simulink model "HybridControllerD3D3_nAct"  (Simulink 7.5)
settings: Solver=FixedStepDiscrete  StartTime=0.0  StopTime=inf  RelTol=1e-3
PreLoadFcn:
  | initializeSimulation
values from neighbouring files (symbols this model uses):
  nAct = 8    [initializeSimulation.m]
  nDout = 4    [initializeSimulation.m]
  node = completenodestruct(node)    [initializeSimulation.m]
undefined symbols (not defined in the file or in its folder): HybridCtrlParameters
libraries: xpclib x14, xpcsystranlib x8, simulink x4
CloseFcn:
  | rtwprivate ssgencode ModelCloseRequest scrnet_receiver
settings Model: Creator=mvetsch  LastModifiedBy=Andreas  ExtModeArmWhenConnect=off  BufferReuse=off
settings DataIOCC: LimitDataPoints=off  SaveOutput=off  SignalLogging=off  SaveTime=off  SignalLoggingName=sigsOut
settings OptimizationCC: BlockReduction=off  OptimizeBlockIOStorage=off  BufferReuse=off  EnforceIntegerDowncast=off  ExpressionFolding=off  FoldNonRolledExpr=off  LocalBlockOutputs=off  StateBitsets=on  DataBitsets=on  UseTempVars=on  InitFltsAndDblsToZero=on  EfficientFloat2IntCast=on  SimCompilerOptimization=On
settings DebuggingCC: SaveWithParameterizedLinksMsg=none  CheckSSInitialOutputMsg=off  SolverPrmCheckMsg=none  StrictBusMsg=None
settings HardwareCC: ProdIntDivRoundTo=Zero  ProdEndianess=LittleEndian  ProdHWDeviceType=Generic->32-bit x86 compatible  TargetHWDeviceType=32-bit Generic
settings SFSimCC: SimCustomHeaderCode="#include \"PredictorCorrector.h\""  SimUserSources=PredictorCorrector.c  SimUserIncludeDirs=D:\PredictorCorrector\HybridSimToolbox
settings RTWCC: SystemTargetFile=xpctarget.tlc  TemplateMakefile=xpc_default_tmf  Description=xPC Target  ProcessScript=xpctarget_make_rtw_hook  CustomHeaderCode="#include \"PredictorCorrector.h\""  CustomInclude=D:\PredictorCorrector\HybridSimToolbox  CustomSource=PredictorCorrector.c  IncludeERTFirstTime=on  RTWCompilerOptimization=On
settings xpcTargetCC: TargetFcnLib=ansi_tfl_tmw.mat  TargetFunctionLibrary=ANSI_C  ERTCodeCoverageTool=None  ParMdlRefBuildCompliant=off  PortableWordSizes=off  RL32IRQSourceModifier=11  xPCIRQSourceBoard=Scramnet_SC150+  xPCLoadParamSetFile=off

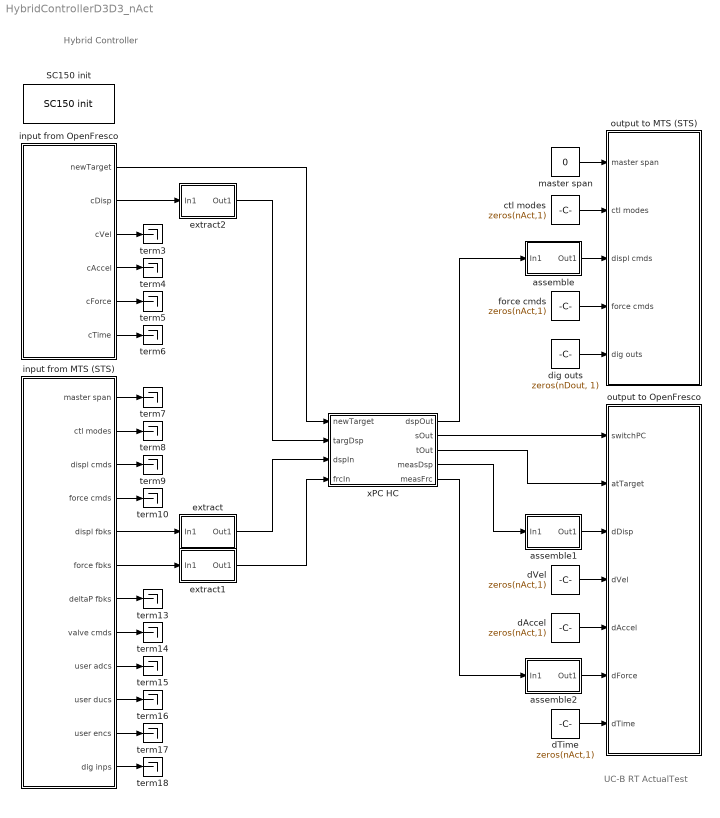
== system HybridControllerD3D3_nAct ==
  note: Hybrid Controller
  note: UC-B RT ActualTest
  SC150 init : xpcsystranlib/Shared Memory/SC150 init   node=node  pci=-1
  assemble : Subsystem  mask(to Actuators){id=[2 3 4 1 5 6], size=nAct}
      mask prompts: id "Index Vector: id"; size "Vector Size: size"
      mask help: To select to which actuator(s) the signals are going to
      mask Display: disp('Assemble')
  assemble1 : Subsystem  mask(to Actuators){id=[2 3 4 1 5 6], size=nAct}
      mask prompts: id "Index Vector: id"; size "Vector Size: size"
      mask help: To select to which actuator(s) the signals are going to
      mask Display: disp('Assemble')
  assemble2 : Subsystem  mask(to Actuators){id=[2 3 4 1 5 6], size=nAct}
      mask prompts: id "Index Vector: id"; size "Vector Size: size"
      mask help: To select to which actuator(s) the signals are going to
      mask Display: disp('Assemble')
  ctl modes : Constant  Value=zeros(nAct,1)  OutDataType=sfix(16)  OutScaling=2^0
  dAccel : Constant  Value=zeros(nAct,1)  OutDataType=sfix(16)  OutScaling=2^0
  dTime : Constant  Value=zeros(nAct,1)  OutDataType=sfix(16)  OutScaling=2^0
  dVel : Constant  Value=zeros(nAct,1)  OutDataType=sfix(16)  OutScaling=2^0
  dig outs : Constant  Value=zeros(nDout, 1)  OutDataTypeMode=uint32  OutDataType=sfix(16)  OutScaling=2^0  OutDataTypeStr=uint32
  extract : Subsystem  mask(from Actuators){id=[2 3 4 1 5 6], size=nAct}
      mask prompts: id "Index Vector: id"; size "Vector Size: size"
      mask help: To select from which actuator(s) the signals are coming from
      mask Display: disp('Extract')
  extract1 : Subsystem  mask(from Actuators){id=[2 3 4 1 5 6], size=nAct}
      mask prompts: id "Index Vector: id"; size "Vector Size: size"
      mask help: To select from which actuator(s) the signals are coming from
      mask Display: disp('Extract')
  extract2 : Subsystem  mask(from Actuators){id=[2 3 4 1 5 6], size=nAct}
      mask prompts: id "Index Vector: id"; size "Vector Size: size"
      mask help: To select from which actuator(s) the signals are coming from
      mask Display: disp('Extract')
  force cmds : Constant  Value=zeros(nAct,1)  OutDataType=sfix(16)  OutScaling=2^0
  input from MTS (STS) : Subsystem
  input from OpenFresco : Subsystem
  master span : Constant  Value=0  OutDataType=sfix(16)  OutScaling=2^0
  output to MTS (STS) : Subsystem
  output to OpenFresco : Subsystem
  term{3..10,13..18} (14 alike) : Terminator
  xPC HC : Subsystem  mask(Hybrid Controller: D3/D3){nAct=6, dtInt=HybridCtrlParameters.dtInt, dtSim=HybridCtrlParameters.dtSim, dtCon=HybridCtrlParameters.dtCon, N=HybridCtrlParameters.N, iDelay=HybridCtrlParameters.iDelay}
      mask prompts: nAct "Number of Actuators: nAct"; dtInt "Integration time step: dtInt"; dtSim "Simulation time step: dtSim"; dtCon "Controller time step: dtCon"; N "Maximum number of substeps: N"; iDelay "Number of delay steps: iDelay"
      mask help: Hybrid Controller using C0-continuous cubic Lagrange interpolation for prediction and correction
      mask Display: disp('xPC Target\nHybrid Controller\n(D3/D3)')
  wires:
  input from MTS (STS)/10(user ducs) -> term16/1
  input from MTS (STS)/12(dig inps) -> term18/1
  input from MTS (STS)/2(ctl modes) -> term8/1
  input from MTS (STS)/4(force cmds) -> term10/1
  input from MTS (STS)/8(valve cmds) -> term14/1
  input from MTS (STS)/1(master span) -> term7/1
  input from MTS (STS)/7(deltaP fbks) -> term13/1
  input from MTS (STS)/9(user adcs) -> term15/1
  input from MTS (STS)/11(user encs) -> term17/1
  master span/1 -> output to MTS (STS)/1(master span)
  force cmds/1 -> output to MTS (STS)/4(force cmds)
  ctl modes/1 -> output to MTS (STS)/2(ctl modes)
  input from MTS (STS)/3(displ cmds) -> term9/1
  input from MTS (STS)/5(displ fbks) -> extract/1(In1)
  dig outs/1 -> output to MTS (STS)/5(dig outs)
  input from MTS (STS)/6(force fbks) -> extract1/1(In1)
  dVel/1 -> output to OpenFresco/4(dVel)
  dAccel/1 -> output to OpenFresco/5(dAccel)
  dTime/1 -> output to OpenFresco/7(dTime)
  input from OpenFresco/3(cVel) -> term3/1
  input from OpenFresco/4(cAccel) -> term4/1
  input from OpenFresco/5(cForce) -> term5/1
  input from OpenFresco/6(cTime) -> term6/1
  assemble/1(Out1) -> output to MTS (STS)/3(displ cmds)
  input from OpenFresco/2(cDisp) -> extract2/1(In1)
  input from OpenFresco/1(newTarget) -> xPC HC/1(newTarget)
  extract2/1(Out1) -> xPC HC/2(targDsp)
  extract/1(Out1) -> xPC HC/3(dspIn)
  extract1/1(Out1) -> xPC HC/4(frcIn)
  xPC HC/1(dspOut) -> assemble/1(In1)
  xPC HC/5(measFrc) -> assemble2/1(In1)
  xPC HC/4(measDsp) -> assemble1/1(In1)
  xPC HC/3(tOut) -> output to OpenFresco/2(atTarget)
  xPC HC/2(sOut) -> output to OpenFresco/1(switchPC)
  assemble1/1(Out1) -> output to OpenFresco/3(dDisp)
  assemble2/1(Out1) -> output to OpenFresco/6(dForce)

== system HybridControllerD3D3_nAct/assemble ==
  In1 : Inport  OutDataType=sfix(16)  OutScaling=2^0
  Assignment : Assignment  OutputInitialize=Specify size for each dimension in table  IndexOptions=Index vector (port)  Indices=1  OutputSizes=nAct
  Constant : Constant  Value=id  OutDataType=sfix(16)  OutScaling=2^0
  Out1 : Outport  OutDataType=sfix(16)  OutScaling=2^0
  wires:
  Constant/1 -> Assignment/2
  Assignment/1 -> Out1/1
  In1/1 -> Assignment/1

== system HybridControllerD3D3_nAct/assemble1 ==
  In1 : Inport  OutDataType=sfix(16)  OutScaling=2^0
  Assignment : Assignment  OutputInitialize=Specify size for each dimension in table  IndexOptions=Index vector (port)  Indices=1  OutputSizes=nAct
  Constant : Constant  Value=id  OutDataType=sfix(16)  OutScaling=2^0
  Out1 : Outport  OutDataType=sfix(16)  OutScaling=2^0
  wires:
  Constant/1 -> Assignment/2
  Assignment/1 -> Out1/1
  In1/1 -> Assignment/1

== system HybridControllerD3D3_nAct/assemble2 ==
  In1 : Inport  OutDataType=sfix(16)  OutScaling=2^0
  Assignment : Assignment  OutputInitialize=Specify size for each dimension in table  IndexOptions=Index vector (port)  Indices=1  OutputSizes=nAct
  Constant : Constant  Value=id  OutDataType=sfix(16)  OutScaling=2^0
  Out1 : Outport  OutDataType=sfix(16)  OutScaling=2^0
  wires:
  Constant/1 -> Assignment/2
  Assignment/1 -> Out1/1
  In1/1 -> Assignment/1

== system HybridControllerD3D3_nAct/extract ==
  In1 : Inport  OutDataType=sfix(16)  OutScaling=2^0
  Selector : Selector  InputPortWidth=size  IndexOptions=Index vector (dialog)  Indices=id  OutputSizes=1
  Out1 : Outport  OutDataType=sfix(16)  OutScaling=2^0
  wires:
  Selector/1 -> Out1/1
  In1/1 -> Selector/1

== system HybridControllerD3D3_nAct/extract1 ==
  In1 : Inport  OutDataType=sfix(16)  OutScaling=2^0
  Selector : Selector  InputPortWidth=size  IndexOptions=Index vector (dialog)  Indices=id  OutputSizes=1
  Out1 : Outport  OutDataType=sfix(16)  OutScaling=2^0
  wires:
  Selector/1 -> Out1/1
  In1/1 -> Selector/1

== system HybridControllerD3D3_nAct/extract2 ==
  In1 : Inport  OutDataType=sfix(16)  OutScaling=2^0
  Selector : Selector  InputPortWidth=size  IndexOptions=Index vector (dialog)  Indices=id  OutputSizes=1
  Out1 : Outport  OutDataType=sfix(16)  OutScaling=2^0
  wires:
  Selector/1 -> Out1/1
  In1/1 -> Selector/1

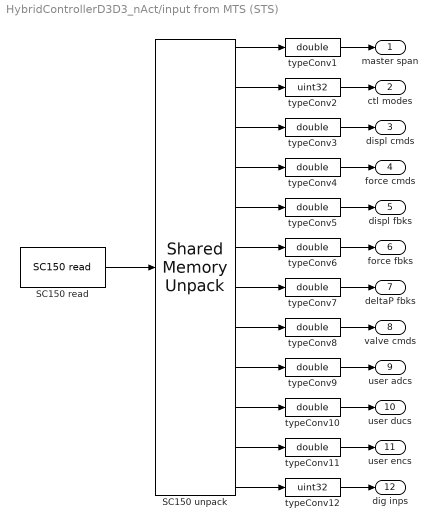
== system HybridControllerD3D3_nAct/input from MTS (STS) ==
  SC150 read : xpcsystranlib/Shared Memory/SC150 read   partition=node.Partitions(12:23)  errorport=off  ts=samplePeriod  pci=-1
  SC150 unpack : xpclib/Shared Memory/Shared Memory Unpack   partition=node.Partitions(12:23)
  typeConv{1,3..11} (10 alike) : DataTypeConversion  OutDataTypeMode=double  OutDataType=sfix(16)  OutScaling=2^0  OutDataTypeStr=double  SaturateOnIntegerOverflow=on  RndMeth=Zero
  typeConv12 : DataTypeConversion  OutDataTypeMode=uint32  OutDataType=sfix(16)  OutScaling=2^0  OutDataTypeStr=uint32  SaturateOnIntegerOverflow=on  RndMeth=Zero
  typeConv2 : DataTypeConversion  OutDataTypeMode=uint32  OutDataType=sfix(16)  OutScaling=2^0  OutDataTypeStr=uint32  SaturateOnIntegerOverflow=on  RndMeth=Zero
  master span : Outport  OutDataType=sfix(16)  OutScaling=2^0
  ctl modes : Outport  Port=2  OutDataType=sfix(16)  OutScaling=2^0
  displ cmds : Outport  Port=3  OutDataType=sfix(16)  OutScaling=2^0
  force cmds : Outport  Port=4  OutDataType=sfix(16)  OutScaling=2^0
  displ fbks : Outport  Port=5  OutDataType=sfix(16)  OutScaling=2^0
  force fbks : Outport  Port=6  OutDataType=sfix(16)  OutScaling=2^0
  deltaP fbks : Outport  Port=7  OutDataType=sfix(16)  OutScaling=2^0
  valve cmds : Outport  Port=8  OutDataType=sfix(16)  OutScaling=2^0
  user adcs : Outport  Port=9  OutDataType=sfix(16)  OutScaling=2^0
  user ducs : Outport  Port=10  OutDataType=sfix(16)  OutScaling=2^0
  user encs : Outport  Port=11  OutDataType=sfix(16)  OutScaling=2^0
  dig inps : Outport  Port=12  OutDataType=sfix(16)  OutScaling=2^0
  wires:
  typeConv11/1 -> user encs/1
  typeConv10/1 -> user ducs/1
  typeConv12/1 -> dig inps/1
  typeConv9/1 -> user adcs/1
  typeConv8/1 -> valve cmds/1
  typeConv7/1 -> deltaP fbks/1
  typeConv6/1 -> force fbks/1
  typeConv5/1 -> displ fbks/1
  typeConv4/1 -> force cmds/1
  typeConv3/1 -> displ cmds/1
  typeConv1/1 -> master span/1
  SC150 read/1 -> SC150 unpack/1
  typeConv2/1 -> ctl modes/1
  SC150 unpack/1 -> typeConv1/1
  SC150 unpack/2 -> typeConv2/1
  SC150 unpack/3 -> typeConv3/1
  SC150 unpack/4 -> typeConv4/1
  SC150 unpack/5 -> typeConv5/1
  SC150 unpack/6 -> typeConv6/1
  SC150 unpack/7 -> typeConv7/1
  SC150 unpack/8 -> typeConv8/1
  SC150 unpack/9 -> typeConv9/1
  SC150 unpack/10 -> typeConv10/1
  SC150 unpack/11 -> typeConv11/1
  SC150 unpack/12 -> typeConv12/1

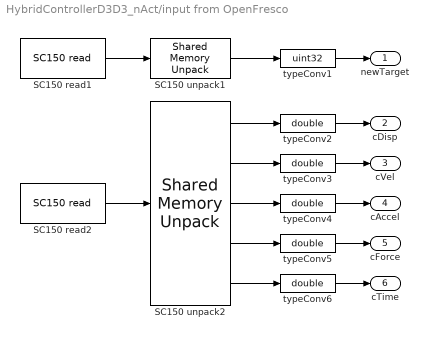
== system HybridControllerD3D3_nAct/input from OpenFresco ==
  SC150 read1 : xpcsystranlib/Shared Memory/SC150 read   partition=node.Partitions(26)  errorport=off  ts=samplePeriod  pci=-1
  SC150 read2 : xpcsystranlib/Shared Memory/SC150 read   partition=node.Partitions(29:33)  errorport=off  ts=samplePeriod  pci=-1
  SC150 unpack1 : xpclib/Shared Memory/Shared Memory Unpack   partition=node.Partitions(26)
  SC150 unpack2 : xpclib/Shared Memory/Shared Memory Unpack   partition=node.Partitions(29:33)
  typeConv1 : DataTypeConversion  OutDataTypeMode=uint32  OutDataType=sfix(16)  OutScaling=2^0  OutDataTypeStr=uint32  SaturateOnIntegerOverflow=on  RndMeth=Zero
  typeConv{2..6} (5 alike) : DataTypeConversion  OutDataTypeMode=double  OutDataType=sfix(16)  OutScaling=2^0  OutDataTypeStr=double  SaturateOnIntegerOverflow=on  RndMeth=Zero
  newTarget : Outport  OutDataType=sfix(16)  OutScaling=2^0
  cDisp : Outport  Port=2  OutDataType=sfix(16)  OutScaling=2^0
  cVel : Outport  Port=3  OutDataType=sfix(16)  OutScaling=2^0
  cAccel : Outport  Port=4  OutDataType=sfix(16)  OutScaling=2^0
  cForce : Outport  Port=5  OutDataType=sfix(16)  OutScaling=2^0
  cTime : Outport  Port=6  OutDataType=sfix(16)  OutScaling=2^0
  wires:
  typeConv1/1 -> newTarget/1
  SC150 read1/1 -> SC150 unpack1/1
  SC150 unpack1/1 -> typeConv1/1
  typeConv2/1 -> cDisp/1
  SC150 unpack2/1 -> typeConv2/1
  typeConv3/1 -> cVel/1
  SC150 unpack2/2 -> typeConv3/1
  typeConv4/1 -> cAccel/1
  SC150 unpack2/3 -> typeConv4/1
  typeConv5/1 -> cForce/1
  typeConv6/1 -> cTime/1
  SC150 unpack2/5 -> typeConv6/1
  SC150 read2/1 -> SC150 unpack2/1
  SC150 unpack2/4 -> typeConv5/1

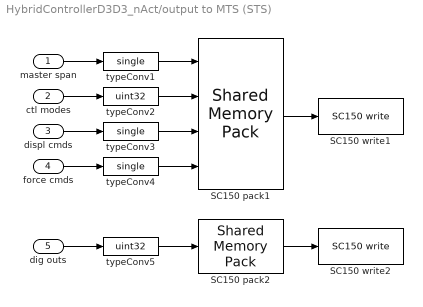
== system HybridControllerD3D3_nAct/output to MTS (STS) ==
  master span : Inport  OutDataType=sfix(16)  OutScaling=2^0
  ctl modes : Inport  Port=2  OutDataType=sfix(16)  OutScaling=2^0
  displ cmds : Inport  Port=3  OutDataType=sfix(16)  OutScaling=2^0
  force cmds : Inport  Port=4  OutDataType=sfix(16)  OutScaling=2^0
  dig outs : Inport  Port=5  OutDataType=sfix(16)  OutScaling=2^0
  SC150 pack1 : xpclib/Shared Memory/Shared Memory Pack   partition=node.Partitions(1:4)
  SC150 pack2 : xpclib/Shared Memory/Shared Memory Pack   partition=node.Partitions(11)
  SC150 write1 : xpcsystranlib/Shared Memory/SC150 write   partition=node.Partitions(1:4)  errorport=off  ts=samplePeriod  pci=-1
  SC150 write2 : xpcsystranlib/Shared Memory/SC150 write   partition=node.Partitions(11)  errorport=off  ts=samplePeriod  pci=-1
  typeConv1 : DataTypeConversion  OutDataTypeMode=single  OutDataType=sfix(16)  OutScaling=2^0  OutDataTypeStr=single  SaturateOnIntegerOverflow=on  RndMeth=Zero
  typeConv2 : DataTypeConversion  OutDataTypeMode=uint32  OutDataType=sfix(16)  OutScaling=2^0  OutDataTypeStr=uint32  SaturateOnIntegerOverflow=on  RndMeth=Zero
  typeConv3 : DataTypeConversion  OutDataTypeMode=single  OutDataType=sfix(16)  OutScaling=2^0  OutDataTypeStr=single  SaturateOnIntegerOverflow=on  RndMeth=Zero
  typeConv4 : DataTypeConversion  OutDataTypeMode=single  OutDataType=sfix(16)  OutScaling=2^0  OutDataTypeStr=single  SaturateOnIntegerOverflow=on  RndMeth=Zero
  typeConv5 : DataTypeConversion  OutDataTypeMode=uint32  OutDataType=sfix(16)  OutScaling=2^0  OutDataTypeStr=uint32  SaturateOnIntegerOverflow=on  RndMeth=Zero
  wires:
  dig outs/1 -> typeConv5/1
  force cmds/1 -> typeConv4/1
  master span/1 -> typeConv1/1
  SC150 pack1/1 -> SC150 write1/1
  displ cmds/1 -> typeConv3/1
  ctl modes/1 -> typeConv2/1
  typeConv1/1 -> SC150 pack1/1
  typeConv2/1 -> SC150 pack1/2
  typeConv3/1 -> SC150 pack1/3
  typeConv4/1 -> SC150 pack1/4
  SC150 pack2/1 -> SC150 write2/1
  typeConv5/1 -> SC150 pack2/1

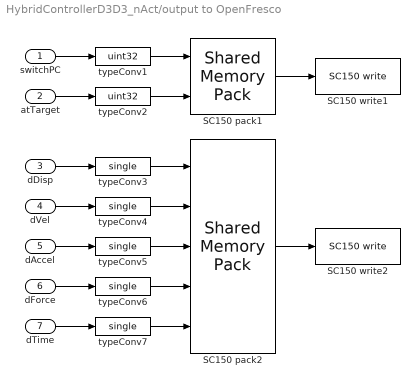
== system HybridControllerD3D3_nAct/output to OpenFresco ==
  switchPC : Inport  OutDataType=sfix(16)  OutScaling=2^0
  atTarget : Inport  Port=2  OutDataType=sfix(16)  OutScaling=2^0
  dDisp : Inport  Port=3  OutDataType=sfix(16)  OutScaling=2^0
  dVel : Inport  Port=4  OutDataType=sfix(16)  OutScaling=2^0
  dAccel : Inport  Port=5  OutDataType=sfix(16)  OutScaling=2^0
  dForce : Inport  Port=6  OutDataType=sfix(16)  OutScaling=2^0
  dTime : Inport  Port=7  OutDataType=sfix(16)  OutScaling=2^0
  SC150 pack1 : xpclib/Shared Memory/Shared Memory Pack   partition=node.Partitions(27:28)
  SC150 pack2 : xpclib/Shared Memory/Shared Memory Pack   partition=node.Partitions(34:38)
  SC150 write1 : xpcsystranlib/Shared Memory/SC150 write   partition=node.Partitions(27:28)  errorport=off  ts=samplePeriod  pci=-1
  SC150 write2 : xpcsystranlib/Shared Memory/SC150 write   partition=node.Partitions(34:38)  errorport=off  ts=samplePeriod  pci=-1
  typeConv1 : DataTypeConversion  OutDataTypeMode=uint32  OutDataType=sfix(16)  OutScaling=2^0  OutDataTypeStr=uint32  SaturateOnIntegerOverflow=on  RndMeth=Zero
  typeConv2 : DataTypeConversion  OutDataTypeMode=uint32  OutDataType=sfix(16)  OutScaling=2^0  OutDataTypeStr=uint32  SaturateOnIntegerOverflow=on  RndMeth=Zero
  typeConv{3..7} (5 alike) : DataTypeConversion  OutDataTypeMode=single  OutDataType=sfix(16)  OutScaling=2^0  OutDataTypeStr=single  SaturateOnIntegerOverflow=on  RndMeth=Zero
  wires:
  dAccel/1 -> typeConv5/1
  switchPC/1 -> typeConv1/1
  SC150 pack1/1 -> SC150 write1/1
  dVel/1 -> typeConv4/1
  dDisp/1 -> typeConv3/1
  typeConv3/1 -> SC150 pack2/1
  typeConv4/1 -> SC150 pack2/2
  typeConv5/1 -> SC150 pack2/3
  dForce/1 -> typeConv6/1
  typeConv6/1 -> SC150 pack2/4
  dTime/1 -> typeConv7/1
  typeConv7/1 -> SC150 pack2/5
  atTarget/1 -> typeConv2/1
  typeConv2/1 -> SC150 pack1/2
  typeConv1/1 -> SC150 pack1/1
  SC150 pack2/1 -> SC150 write2/1

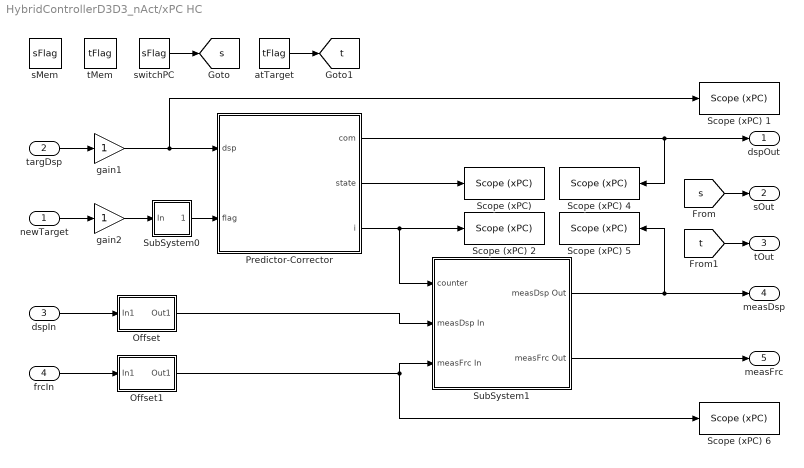
== system HybridControllerD3D3_nAct/xPC HC ==
  newTarget : Inport  OutDataType=sfix(16)  OutScaling=2^0
  targDsp : Inport  Port=2  OutDataType=sfix(16)  OutScaling=2^0
  dspIn : Inport  Port=3  OutDataType=sfix(16)  OutScaling=2^0
  frcIn : Inport  Port=4  OutDataType=sfix(16)  OutScaling=2^0
  Offset : Subsystem  mask(Signal Offset){nS=nAct, nOffset=1024, dt=dtCon}
      mask prompts: nS "Number of Signals: nS"; nOffset "Number of samples to initialize offset: nOffset"; dt "Sample time: dt"
      mask help: Offset signal by average of signal over initial number of samples
      mask Display: fprintf('Signal\nOffset')
  Offset1 : Subsystem  mask(Signal Offset){nS=nAct, nOffset=1024, dt=dtCon}
      mask prompts: nS "Number of Signals: nS"; nOffset "Number of samples to initialize offset: nOffset"; dt "Sample time: dt"
      mask help: Offset signal by average of signal over initial number of samples
      mask Display: fprintf('Signal\nOffset')
  Predictor-Corrector : Stateflow chart  TreatAsAtomicUnit=on
  "Scope (xPC) " : xpclib/Misc./Scope (xPC)   SystemSampleTime=-1  scopeno=4  scopetype=File  autostart=on  viewmode=Graphical redraw  formatstr='%15.6f'  grid=on  ylimits=[0,3]  nosamples=4096  noprepostsamples=0  interleave=1  triggermode=FreeRun  triggersignal=1  triggerlevel=0.0  triggerslope=Either  triggerscope=1  triggersample=0  filename=state.dat  mode=Lazy  writesize=512  autorestart=on  dynamicfilemode=off  maxwritefilesize=512*1024^2
  Scope (xPC) 1 : xpclib/Misc./Scope (xPC)   SystemSampleTime=-1  scopeno=1  scopetype=File  autostart=on  viewmode=Numerical  formatstr='%15.6f'  grid=on  ylimits=[-4,4]  nosamples=4096  noprepostsamples=0  interleave=1  triggermode=FreeRun  triggersignal=1  triggerlevel=0.0  triggerslope=Either  triggerscope=1  triggersample=0  filename=targDsp.dat  mode=Lazy  writesize=512  autorestart=on  dynamicfilemode=off  maxwritefilesize=512*1024^2
  Scope (xPC) 2 : xpclib/Misc./Scope (xPC)   SystemSampleTime=-1  scopeno=5  scopetype=File  autostart=on  viewmode=Numerical  formatstr='%15.6f'  grid=on  ylimits=[0,3]  nosamples=4096  noprepostsamples=0  interleave=1  triggermode=FreeRun  triggersignal=1  triggerlevel=0.0  triggerslope=Either  triggerscope=1  triggersample=0  filename=count.dat  mode=Lazy  writesize=512  autorestart=on  dynamicfilemode=off  maxwritefilesize=512*1024^2
  Scope (xPC) 4 : xpclib/Misc./Scope (xPC)   SystemSampleTime=-1  scopeno=2  scopetype=File  autostart=on  viewmode=Numerical  formatstr='%15.6f'  grid=on  ylimits=[-4,4]  nosamples=4096  noprepostsamples=0  interleave=1  triggermode=FreeRun  triggersignal=1  triggerlevel=0.0  triggerslope=Either  triggerscope=1  triggersample=0  filename=commDsp.dat  mode=Lazy  writesize=512  autorestart=on  dynamicfilemode=off  maxwritefilesize=512*1024^2
  Scope (xPC) 5 : xpclib/Misc./Scope (xPC)   SystemSampleTime=-1  scopeno=3  scopetype=File  autostart=on  viewmode=Numerical  formatstr='%15.6f'  grid=on  ylimits=[-4,4]  nosamples=4096  noprepostsamples=0  interleave=1  triggermode=FreeRun  triggersignal=1  triggerlevel=0.0  triggerslope=Either  triggerscope=1  triggersample=0  filename=measDsp.dat  mode=Lazy  writesize=512  autorestart=on  dynamicfilemode=off  maxwritefilesize=512*1024^2
  Scope (xPC) 6 : xpclib/Misc./Scope (xPC)   SystemSampleTime=-1  scopeno=6  scopetype=File  autostart=on  viewmode=Numerical  formatstr='%15.6f'  grid=on  ylimits=[0,3]  nosamples=4096  noprepostsamples=0  interleave=1  triggermode=FreeRun  triggersignal=1  triggerlevel=0.0  triggerslope=Either  triggerscope=1  triggersample=0  filename=measFrc.dat  mode=Lazy  writesize=512  autorestart=on  dynamicfilemode=off  maxwritefilesize=512*1024^2
  SubSystem0 : Subsystem
  SubSystem1 : Subsystem
  atTarget : DataStoreRead  DataStoreName=tFlag  SampleTime=dtCon
  gain1 : Gain  ParameterDataType=sfix(16)  ParameterScaling=2^0  OutDataType=sfix(16)  OutScaling=2^0
  gain2 : Gain  ParameterDataType=sfix(16)  ParameterScaling=2^0  OutDataType=sfix(16)  OutScaling=2^0  OutDataTypeStr=Inherit: Same as input  ParamDataTypeStr=Inherit: Same as input
  sMem : DataStoreMemory  DataStoreName=sFlag  DataType=uint32  OutDataType=sfix(16)  OutScaling=2^0  OutDataTypeStr=uint32
  switchPC : DataStoreRead  DataStoreName=sFlag  SampleTime=dtCon
  tMem : DataStoreMemory  DataStoreName=tFlag  DataType=uint32  OutDataType=sfix(16)  OutScaling=2^0  OutDataTypeStr=uint32
  dspOut : Outport  OutDataType=sfix(16)  OutScaling=2^0
  sOut : Outport  Port=2  OutDataType=sfix(16)  OutScaling=2^0
  tOut : Outport  Port=3  OutDataType=sfix(16)  OutScaling=2^0
  measDsp : Outport  Port=4  OutDataType=sfix(16)  OutScaling=2^0
  measFrc : Outport  Port=5  OutDataType=sfix(16)  OutScaling=2^0
  tag scope: s=global, t=global
  wires:
  frcIn/1 -> Offset1/1(In1)
  dspIn/1 -> Offset/1(In1)
  SubSystem1/2(measFrc Out) -> measFrc/1
  SubSystem1/1(measDsp Out) -> Scope (xPC) 5/1, measDsp/1
  Predictor-Corrector/3(i) -> SubSystem1/1(counter), Scope (xPC) 2/1
  Predictor-Corrector/2(state) -> "Scope (xPC) "/1
  Predictor-Corrector/1(com) -> dspOut/1, Scope (xPC) 4/1
  Offset/1(Out1) -> SubSystem1/2(measDsp In)
  SubSystem0/1(Out) -> Predictor-Corrector/2(flag)
  newTarget/1 -> gain2/1
  switchPC/1 -> [s]
  atTarget/1 -> [t]
  targDsp/1 -> gain1/1
  Offset1/1(Out1) -> Scope (xPC) 6/1, SubSystem1/3(measFrc In)
  [s] -> sOut/1
  [t] -> tOut/1
  gain1/1 -> Predictor-Corrector/1(dsp), Scope (xPC) 1/1
  gain2/1 -> SubSystem0/1(In)

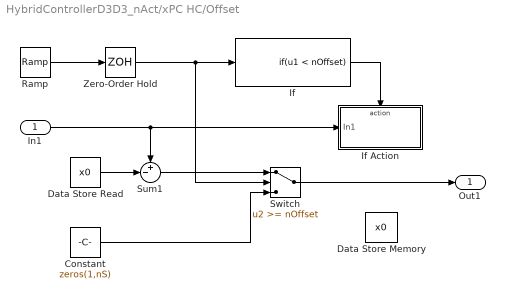
== system HybridControllerD3D3_nAct/xPC HC/Offset ==
  In1 : Inport  OutDataType=sfix(16)  OutScaling=2^0
  Constant : Constant  Value=zeros(1,nS)  OutDataType=sfix(16)  OutScaling=2^0
  Data Store Memory : DataStoreMemory  DataStoreName=x0  InitialValue=zeros(1,nS)  DataType=double  OutDataType=sfix(16)  OutScaling=2^0  OutDataTypeStr=double
  Data Store Read : DataStoreRead  DataStoreName=x0  SampleTime=dt
  If : If  IfExpression=u1 < nOffset  ShowElse=off
  If Action : Subsystem  TreatAsAtomicUnit=on
  Ramp : simulink/Sources/Ramp  SystemSampleTime=-1  slope=1/dt  start=0  X0=0
  Sum1 : Sum  Inputs=+-|  OutDataType=sfix(16)  OutScaling=2^0  SaturateOnIntegerOverflow=on  InputSameDT=on  OutDataTypeStr=Inherit: Same as first input
  Switch : Switch  Threshold=nOffset  SaturateOnIntegerOverflow=on  InputSameDT=on
  Zero-Order Hold : ZeroOrderHold  SampleTime=dt
  Out1 : Outport  OutDataType=sfix(16)  OutScaling=2^0
  wires:
  Switch/1 -> Out1/1
  Sum1/1 -> Switch/1
  Data Store Read/1 -> Sum1/2
  In1/1 -> If Action/1(In1), Sum1/1
  Constant/1 -> Switch/3
  Zero-Order Hold/1 -> Switch/2, If/1
  If/1 -> If Action/Action
  Ramp/1 -> Zero-Order Hold/1

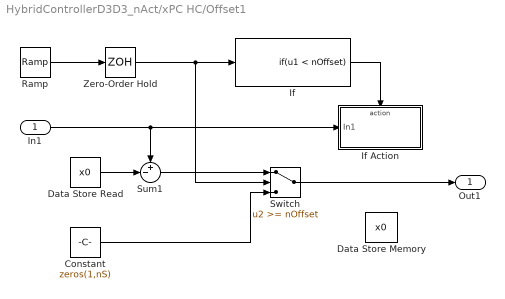
== system HybridControllerD3D3_nAct/xPC HC/Offset1 ==
  In1 : Inport  OutDataType=sfix(16)  OutScaling=2^0
  Constant : Constant  Value=zeros(1,nS)  OutDataType=sfix(16)  OutScaling=2^0
  Data Store Memory : DataStoreMemory  DataStoreName=x0  InitialValue=zeros(1,nS)  DataType=double  OutDataType=sfix(16)  OutScaling=2^0  OutDataTypeStr=double
  Data Store Read : DataStoreRead  DataStoreName=x0  SampleTime=dt
  If : If  IfExpression=u1 < nOffset  ShowElse=off
  If Action : Subsystem  TreatAsAtomicUnit=on
  Ramp : simulink/Sources/Ramp  SystemSampleTime=-1  slope=1/dt  start=0  X0=0
  Sum1 : Sum  Inputs=+-|  OutDataType=sfix(16)  OutScaling=2^0  SaturateOnIntegerOverflow=on  InputSameDT=on  OutDataTypeStr=Inherit: Same as first input
  Switch : Switch  Threshold=nOffset  SaturateOnIntegerOverflow=on  InputSameDT=on
  Zero-Order Hold : ZeroOrderHold  SampleTime=dt
  Out1 : Outport  OutDataType=sfix(16)  OutScaling=2^0
  wires:
  Switch/1 -> Out1/1
  Sum1/1 -> Switch/1
  Data Store Read/1 -> Sum1/2
  In1/1 -> If Action/1(In1), Sum1/1
  Constant/1 -> Switch/3
  Zero-Order Hold/1 -> Switch/2, If/1
  If/1 -> If Action/Action
  Ramp/1 -> Zero-Order Hold/1

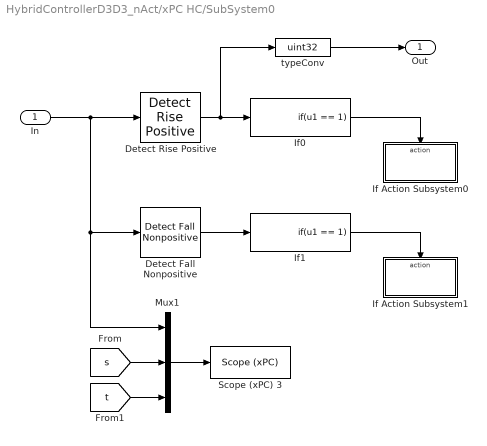
== system HybridControllerD3D3_nAct/xPC HC/SubSystem0 ==
  In : Inport  OutDataType=sfix(16)  OutScaling=2^0
  Detect Fall Nonpositive : simulink/Logic and Bit Operations/Detect Fall Nonpositive  SystemSampleTime=-1  vinit=0
  Detect Rise Positive : simulink/Logic and Bit Operations/Detect Rise Positive  SystemSampleTime=-1  vinit=0
  If Action Subsystem0 : Subsystem  TreatAsAtomicUnit=on
  If Action Subsystem1 : Subsystem  TreatAsAtomicUnit=on
  If0 : If  IfExpression=u1 == 1  ShowElse=off
  If1 : If  IfExpression=u1 == 1  ShowElse=off
  Mux1 : Mux  Inputs=3
  Scope (xPC) 3 : xpclib/Misc./Scope (xPC)   SystemSampleTime=-1  scopeno=7  scopetype=File  autostart=on  viewmode=Numerical  formatstr='%15.6f'  grid=on  ylimits=[0,3]  nosamples=4096  noprepostsamples=0  interleave=1  triggermode=FreeRun  triggersignal=1  triggerlevel=0.0  triggerslope=Either  triggerscope=1  triggersample=0  filename=flag.dat  mode=Lazy  writesize=512  autorestart=on  dynamicfilemode=off  maxwritefilesize=512*1024^2
  typeConv : DataTypeConversion  OutDataTypeMode=uint32  OutDataType=sfix(16)  OutScaling=2^0  OutDataTypeStr=uint32  SaturateOnIntegerOverflow=on  RndMeth=Zero
  Out : Outport  OutDataType=sfix(16)  OutScaling=2^0
  wires:
  In/1 -> Detect Rise Positive/1, Detect Fall Nonpositive/1, Mux1/1
  Detect Rise Positive/1 -> If0/1, typeConv/1
  Detect Fall Nonpositive/1 -> If1/1
  If1/1 -> If Action Subsystem1/Action
  If0/1 -> If Action Subsystem0/Action
  typeConv/1 -> Out/1
  Mux1/1 -> Scope (xPC) 3/1
  [s] -> Mux1/2
  [t] -> Mux1/3

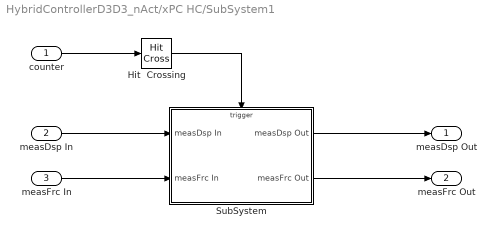
== system HybridControllerD3D3_nAct/xPC HC/SubSystem1 ==
  counter : Inport  OutDataType=sfix(16)  OutScaling=2^0
  measDsp In : Inport  Port=2  OutDataType=sfix(16)  OutScaling=2^0
  measFrc In : Inport  Port=3  OutDataType=sfix(16)  OutScaling=2^0
  Hit  Crossing : HitCross  HitCrossingOffset=iDelay  HitCrossingDirection=rising
  SubSystem : Subsystem  TreatAsAtomicUnit=on
  measDsp Out : Outport  OutDataType=sfix(16)  OutScaling=2^0
  measFrc Out : Outport  Port=2  OutDataType=sfix(16)  OutScaling=2^0
  wires:
  SubSystem/2(measFrc Out) -> measFrc Out/1
  measFrc In/1 -> SubSystem/2(measFrc In)
  SubSystem/1(measDsp Out) -> measDsp Out/1
  measDsp In/1 -> SubSystem/1(measDsp In)
  counter/1 -> Hit  Crossing/1
  Hit  Crossing/1 -> SubSystem/Trigger

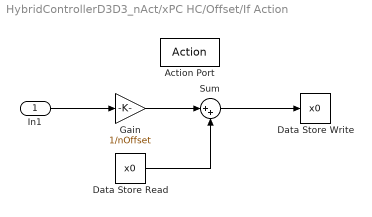
== system HybridControllerD3D3_nAct/xPC HC/Offset/If Action ==
  In1 : Inport  OutDataType=sfix(16)  OutScaling=2^0
  Action Port : ActionPort  PropagateVarSize=During execution
  Data Store Read : DataStoreRead  DataStoreName=x0  SampleTime=dt
  Data Store Write : DataStoreWrite  DataStoreName=x0  SampleTime=-1
  Gain : Gain  Gain=1/nOffset  ParameterDataType=sfix(16)  ParameterScaling=2^0  OutDataType=sfix(16)  OutScaling=2^0  SaturateOnIntegerOverflow=on  OutDataTypeStr=Inherit: Same as input  ParamDataTypeStr=Inherit: Same as input
  Sum : Sum  Inputs=|++  OutDataType=sfix(16)  OutScaling=2^0  SaturateOnIntegerOverflow=on  InputSameDT=on  OutDataTypeStr=Inherit: Same as first input
  wires:
  Data Store Read/1 -> Sum/2
  Sum/1 -> Data Store Write/1
  Gain/1 -> Sum/1
  In1/1 -> Gain/1

== system HybridControllerD3D3_nAct/xPC HC/Offset1/If Action ==
  In1 : Inport  OutDataType=sfix(16)  OutScaling=2^0
  Action Port : ActionPort  PropagateVarSize=During execution
  Data Store Read : DataStoreRead  DataStoreName=x0  SampleTime=dt
  Data Store Write : DataStoreWrite  DataStoreName=x0  SampleTime=-1
  Gain : Gain  Gain=1/nOffset  ParameterDataType=sfix(16)  ParameterScaling=2^0  OutDataType=sfix(16)  OutScaling=2^0  SaturateOnIntegerOverflow=on  OutDataTypeStr=Inherit: Same as input  ParamDataTypeStr=Inherit: Same as input
  Sum : Sum  Inputs=|++  OutDataType=sfix(16)  OutScaling=2^0  SaturateOnIntegerOverflow=on  InputSameDT=on  OutDataTypeStr=Inherit: Same as first input
  wires:
  Data Store Read/1 -> Sum/2
  Sum/1 -> Data Store Write/1
  Gain/1 -> Sum/1
  In1/1 -> Gain/1

== system HybridControllerD3D3_nAct/xPC HC/SubSystem0/If Action Subsystem0 ==
  Action Port : ActionPort  PropagateVarSize=During execution  ActionType=then
  Data Store Write0 : DataStoreWrite  DataStoreName=sFlag  SampleTime=-1
  Data Store Write1 : DataStoreWrite  DataStoreName=tFlag  SampleTime=-1
  atTargetFlag : Constant  Value=0  OutDataTypeMode=uint32  OutDataType=sfix(16)  OutScaling=2^0  OutDataTypeStr=uint32  SampleTime=dtCon
  switchFlag : Constant  OutDataTypeMode=uint32  OutDataType=sfix(16)  OutScaling=2^0  OutDataTypeStr=uint32  SampleTime=dtCon
  wires:
  atTargetFlag/1 -> Data Store Write1/1
  switchFlag/1 -> Data Store Write0/1

== system HybridControllerD3D3_nAct/xPC HC/SubSystem0/If Action Subsystem1 ==
  Action Port : ActionPort  PropagateVarSize=During execution  ActionType=then
  Data Store Write0 : DataStoreWrite  DataStoreName=sFlag  SampleTime=-1
  switchFlag : Constant  Value=0  OutDataTypeMode=uint32  OutDataType=sfix(16)  OutScaling=2^0  OutDataTypeStr=uint32  SampleTime=dtCon
  wires:
  switchFlag/1 -> Data Store Write0/1

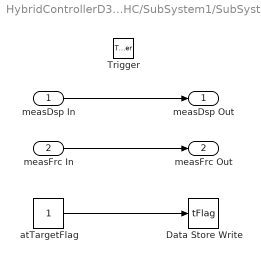
== system HybridControllerD3D3_nAct/xPC HC/SubSystem1/SubSystem ==
  measDsp In : Inport  OutDataType=sfix(16)  OutScaling=2^0
  measFrc In : Inport  Port=2  OutDataType=sfix(16)  OutScaling=2^0
  Trigger : TriggerPort
  Data Store Write : DataStoreWrite  DataStoreName=tFlag  SampleTime=-1
  atTargetFlag : Constant  OutDataTypeMode=uint32  OutDataType=sfix(16)  OutScaling=2^0  OutDataTypeStr=uint32  SampleTime=-1
  measDsp Out : Outport  OutDataType=sfix(16)  OutScaling=2^0  InitialOutput=[0]
  measFrc Out : Outport  Port=2  OutDataType=sfix(16)  OutScaling=2^0  InitialOutput=[0]
  wires:
  atTargetFlag/1 -> Data Store Write/1
  measFrc In/1 -> measFrc Out/1
  measDsp In/1 -> measDsp Out/1

== stateflow chart xPC HC/Predictor-Corrector ==
  state HybridController [parallel]
    settings: executionOrder=1
    state Predict
      en: state = 1;
      en: diSD = 1;
      en: i = 1; iSD = 0;
      en: predictD3(com,i/N);
      du: i++;
      du: predictD3(com,i/N);
    state Initialize
      en: i = 1; iSD = 0;
      en: diSD = 1;
      en: initData(nAct,dtCon);
      en: zeroDsp(com);
    state AutoSlowDown
      en: state = 2;
      en: diSD = 4-i/(0.2*N);
      en: i += diSD; iSD = i;
      en: predictD3(com,i/N);
      du: diSD = 4-i/(0.2*N);
      du: i += diSD; iSD = i;
      du: predictD3(com,i/N);
    state Correct
      en: state = 0;
      en: setCurDsp(com,i/N);
      en: dspLocal = dsp; setNewDsp(dspLocal);
      en: di = min(max(diSD+1/(0.2*N)*(i-iSD),0.001),1.0);
      en: i = min(i+di,N);
      en: correctD3(com,i/N);
      du: di = min(max(diSD+1/(0.2*N)*(i-iSD),0.001),1.0);
      du: i = min(i+di,N);
      du: correctD3(com,i/N);
    Correct -> Predict : [i>=N]
    (default) -> Initialize
    Predict -> Correct [order 2] : [flag==1]
    Initialize -> Correct : [flag==1]
    AutoSlowDown -> Correct : [flag==1]
    Predict -> AutoSlowDown [order 1] : [i>=0.6*N && flag~=1]
  data: dsp input double size=nAct; flag input uint32 size=1; com output double size=nAct; state output uint32 size=1; i output double size=1; N local double size=1; nAct parameter uint32 size=1 =1; iDelay local double size=1; di local double size=1; diSD local double size=1; iSD local double size=1; dspLocal local double size=nAct
